simulink model "LFMT_System_Connection"  (R2026a)
settings: Solver=FixedStepAuto  StopTime=15.0  FixedStep=0.04
libraries: simulink x2
settings Model: Creator=Lenovo  LastModifiedBy=Lenovo

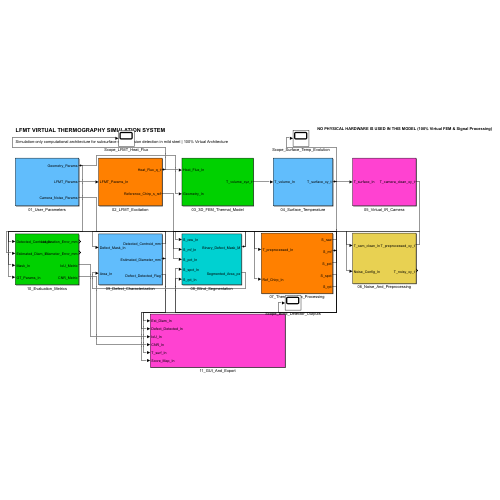
[thumbnail: Simulink's stored preview of the top-level diagram]
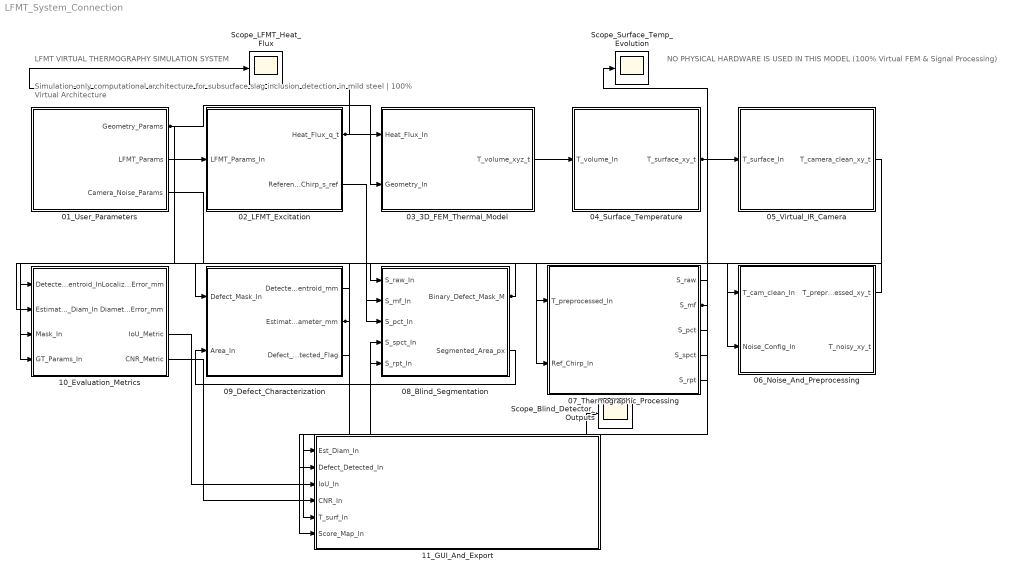
== system LFMT_System_Connection ==
  note: LFMT VIRTUAL THERMOGRAPHY SIMULATION SYSTEM
  note: Simulation-only computational architecture for subsurface slag inclusion detection in mild steel | 100% Virtual Architecture
  note: NO PHYSICAL HARDWARE IS USED IN THIS MODEL (100% Virtual FEM & Signal Processing)
  01_User_Parameters : Subsystem
  02_LFMT_Excitation : Subsystem
  03_3D_FEM_Thermal_Model : Subsystem
  04_Surface_Temperature : Subsystem
  05_Virtual_IR_Camera : Subsystem
  06_Noise_And_Preprocessing : Subsystem
  07_Thermographic_Processing : Subsystem
  08_Blind_Segmentation : Subsystem
  09_Defect_Characterization : Subsystem
  10_Evaluation_Metrics : Subsystem
  11_GUI_And_Export : Subsystem
  Scope_Blind_Detector_Outputs : Scope
  Scope_LFMT_Heat_Flux : Scope
  Scope_Surface_Temp_Evolution : Scope
  wires:
  01_User_Parameters/2(LFMT_Params) -> 02_LFMT_Excitation/1(LFMT_Params_In)
  01_User_Parameters/1(Geometry_Params) -> 03_3D_FEM_Thermal_Model/2(Geometry_In), 10_Evaluation_Metrics/4(GT_Params_In)
  01_User_Parameters/3(Camera_Noise_Params) -> 06_Noise_And_Preprocessing/2(Noise_Config_In)
  02_LFMT_Excitation/1(Heat_Flux_q_t) -> 03_3D_FEM_Thermal_Model/1(Heat_Flux_In), Scope_LFMT_Heat_Flux/1
  02_LFMT_Excitation/2(Reference_Chirp_s_ref) -> 07_Thermographic_Processing/2(Ref_Chirp_In)
  03_3D_FEM_Thermal_Model/1(T_volume_xyz_t) -> 04_Surface_Temperature/1(T_volume_In)
  04_Surface_Temperature/1(T_surface_xy_t) -> 05_Virtual_IR_Camera/1(T_surface_In), Scope_Surface_Temp_Evolution/1, 11_GUI_And_Export/5(T_surf_In)
  05_Virtual_IR_Camera/1(T_camera_clean_xy_t) -> 06_Noise_And_Preprocessing/1(T_cam_clean_In)
  06_Noise_And_Preprocessing/1(T_preprocessed_xy_t) -> 07_Thermographic_Processing/1(T_preprocessed_In)
  07_Thermographic_Processing/1(S_raw) -> 08_Blind_Segmentation/1(S_raw_In)
  07_Thermographic_Processing/2(S_mf) -> 08_Blind_Segmentation/2(S_mf_In), Scope_Blind_Detector_Outputs/1, 11_GUI_And_Export/6(Score_Map_In)
  07_Thermographic_Processing/3(S_pct) -> 08_Blind_Segmentation/3(S_pct_In)
  07_Thermographic_Processing/4(S_spct) -> 08_Blind_Segmentation/4(S_spct_In)
  07_Thermographic_Processing/5(S_rpt) -> 08_Blind_Segmentation/5(S_rpt_In)
  08_Blind_Segmentation/1(Binary_Defect_Mask_M) -> 09_Defect_Characterization/1(Defect_Mask_In), 10_Evaluation_Metrics/3(Mask_In)
  08_Blind_Segmentation/2(Segmented_Area_px) -> 09_Defect_Characterization/2(Area_In)
  09_Defect_Characterization/1(Detected_Centroid_mm) -> 10_Evaluation_Metrics/1(Detected_Centroid_In)
  09_Defect_Characterization/2(Estimated_Diameter_mm) -> 10_Evaluation_Metrics/2(Estimated_Diam_In), 11_GUI_And_Export/1(Est_Diam_In)
  09_Defect_Characterization/3(Defect_Detected_Flag) -> 11_GUI_And_Export/2(Defect_Detected_In)
  10_Evaluation_Metrics/3(IoU_Metric) -> 11_GUI_And_Export/3(IoU_In)
  10_Evaluation_Metrics/4(CNR_Metric) -> 11_GUI_And_Export/4(CNR_In)

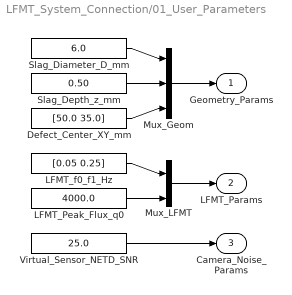
== system LFMT_System_Connection/01_User_Parameters ==
  Defect_Center_XY_mm : Constant  Value=[50.0 35.0]
  LFMT_Peak_Flux_q0 : Constant  Value=4000.0
  LFMT_f0_f1_Hz : Constant  Value=[0.05 0.25]
  Mux_Geom : Mux  Inputs=3
  Mux_LFMT : Mux  Inputs=2
  Slag_Depth_z_mm : Constant  Value=0.50
  Slag_Diameter_D_mm : Constant  Value=6.0
  Virtual_Sensor_NETD_SNR : Constant  Value=25.0
  Geometry_Params : Outport
  LFMT_Params : Outport  Port=2
  Camera_Noise_Params : Outport  Port=3
  wires:
  Slag_Diameter_D_mm/1 -> Mux_Geom/1
  Slag_Depth_z_mm/1 -> Mux_Geom/2
  Defect_Center_XY_mm/1 -> Mux_Geom/3
  Mux_Geom/1 -> Geometry_Params/1
  LFMT_f0_f1_Hz/1 -> Mux_LFMT/1
  LFMT_Peak_Flux_q0/1 -> Mux_LFMT/2
  Mux_LFMT/1 -> LFMT_Params/1
  Virtual_Sensor_NETD_SNR/1 -> Camera_Noise_Params/1

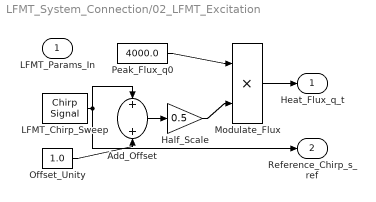
== system LFMT_System_Connection/02_LFMT_Excitation ==
  LFMT_Params_In : Inport
  Add_Offset : Sum
  Half_Scale : Gain  Gain=0.5
  LFMT_Chirp_Sweep : simulink/Sources/Chirp Signal  f1=0.05  T=10.0  f2=0.25
  Modulate_Flux : Product
  Offset_Unity : Constant  Value=1.0
  Peak_Flux_q0 : Constant  Value=4000.0
  Heat_Flux_q_t : Outport
  Reference_Chirp_s_ref : Outport  Port=2
  wires:
  LFMT_Chirp_Sweep/1 -> Add_Offset/1, Reference_Chirp_s_ref/1
  Offset_Unity/1 -> Add_Offset/2
  Add_Offset/1 -> Half_Scale/1
  Peak_Flux_q0/1 -> Modulate_Flux/1
  Half_Scale/1 -> Modulate_Flux/2
  Modulate_Flux/1 -> Heat_Flux_q_t/1

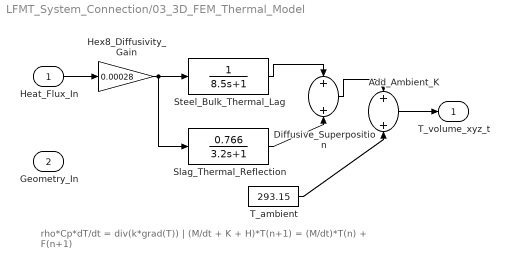
== system LFMT_System_Connection/03_3D_FEM_Thermal_Model ==
  note: rho*Cp*dT/dt = div(k*grad(T)) | (M/dt + K + H)*T(n+1) = (M/dt)*T(n) + F(n+1)
  Heat_Flux_In : Inport
  Geometry_In : Inport  Port=2
  Add_Ambient_K : Sum
  Diffusive_Superposition : Sum
  Hex8_Diffusivity_Gain : Gain  Gain=0.00028
  Slag_Thermal_Reflection : TransferFcn  Numerator=[0.766]  Denominator=[3.2 1]
  Steel_Bulk_Thermal_Lag : TransferFcn  Denominator=[8.5 1]
  T_ambient : Constant  Value=293.15
  T_volume_xyz_t : Outport
  wires:
  Heat_Flux_In/1 -> Hex8_Diffusivity_Gain/1
  Hex8_Diffusivity_Gain/1 -> Steel_Bulk_Thermal_Lag/1, Slag_Thermal_Reflection/1
  Steel_Bulk_Thermal_Lag/1 -> Diffusive_Superposition/1
  Slag_Thermal_Reflection/1 -> Diffusive_Superposition/2
  Diffusive_Superposition/1 -> Add_Ambient_K/1
  T_ambient/1 -> Add_Ambient_K/2
  Add_Ambient_K/1 -> T_volume_xyz_t/1

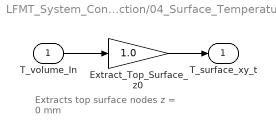
== system LFMT_System_Connection/04_Surface_Temperature ==
  note: Extracts top surface nodes z = 0 mm
  T_volume_In : Inport
  Extract_Top_Surface_z0 : Gain  Gain=1.0
  T_surface_xy_t : Outport
  wires:
  T_volume_In/1 -> Extract_Top_Surface_z0/1
  Extract_Top_Surface_z0/1 -> T_surface_xy_t/1

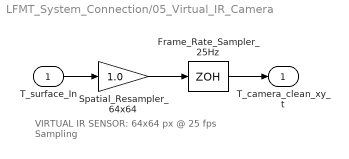
== system LFMT_System_Connection/05_Virtual_IR_Camera ==
  note: VIRTUAL IR SENSOR: 64x64 px @ 25 fps Sampling
  T_surface_In : Inport
  Frame_Rate_Sampler_25Hz : ZeroOrderHold  SampleTime=0.04
  Spatial_Resampler_64x64 : Gain  Gain=1.0
  T_camera_clean_xy_t : Outport
  wires:
  T_surface_In/1 -> Spatial_Resampler_64x64/1
  Spatial_Resampler_64x64/1 -> Frame_Rate_Sampler_25Hz/1
  Frame_Rate_Sampler_25Hz/1 -> T_camera_clean_xy_t/1

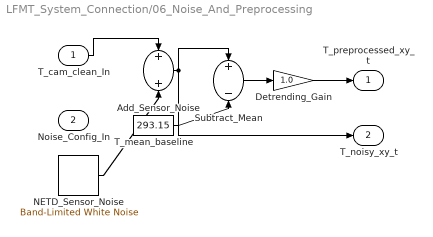
== system LFMT_System_Connection/06_Noise_And_Preprocessing ==
  T_cam_clean_In : Inport
  Noise_Config_In : Inport  Port=2
  Add_Sensor_Noise : Sum
  Detrending_Gain : Gain  Gain=1.0
  NETD_Sensor_Noise : simulink/Sources/Band-Limited White Noise  Cov=0.0004  Ts=0.04  seed=[23341]
  Subtract_Mean : Sum  Inputs=+-
  T_mean_baseline : Constant  Value=293.15
  T_preprocessed_xy_t : Outport
  T_noisy_xy_t : Outport  Port=2
  wires:
  T_cam_clean_In/1 -> Add_Sensor_Noise/1
  NETD_Sensor_Noise/1 -> Add_Sensor_Noise/2
  Add_Sensor_Noise/1 -> Subtract_Mean/1, T_noisy_xy_t/1
  T_mean_baseline/1 -> Subtract_Mean/2
  Subtract_Mean/1 -> Detrending_Gain/1
  Detrending_Gain/1 -> T_preprocessed_xy_t/1

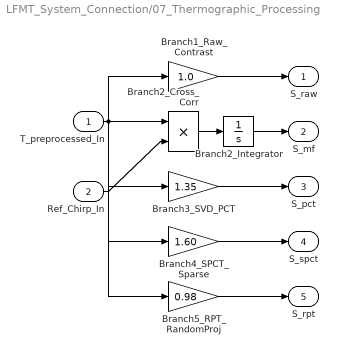
== system LFMT_System_Connection/07_Thermographic_Processing ==
  T_preprocessed_In : Inport
  Ref_Chirp_In : Inport  Port=2
  Branch1_Raw_Contrast : Gain  Gain=1.0
  Branch2_Cross_Corr : Product
  Branch2_Integrator : Integrator
  Branch3_SVD_PCT : Gain  Gain=1.35
  Branch4_SPCT_Sparse : Gain  Gain=1.60
  Branch5_RPT_RandomProj : Gain  Gain=0.98
  S_raw : Outport
  S_mf : Outport  Port=2
  S_pct : Outport  Port=3
  S_spct : Outport  Port=4
  S_rpt : Outport  Port=5
  wires:
  T_preprocessed_In/1 -> Branch1_Raw_Contrast/1, Branch2_Cross_Corr/1, Branch3_SVD_PCT/1, Branch4_SPCT_Sparse/1, Branch5_RPT_RandomProj/1
  Branch1_Raw_Contrast/1 -> S_raw/1
  Ref_Chirp_In/1 -> Branch2_Cross_Corr/2
  Branch2_Cross_Corr/1 -> Branch2_Integrator/1
  Branch2_Integrator/1 -> S_mf/1
  Branch3_SVD_PCT/1 -> S_pct/1
  Branch4_SPCT_Sparse/1 -> S_spct/1
  Branch5_RPT_RandomProj/1 -> S_rpt/1

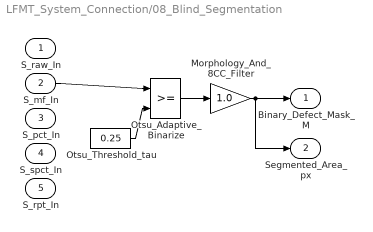
== system LFMT_System_Connection/08_Blind_Segmentation ==
  S_raw_In : Inport
  S_mf_In : Inport  Port=2
  S_pct_In : Inport  Port=3
  S_spct_In : Inport  Port=4
  S_rpt_In : Inport  Port=5
  Morphology_And_8CC_Filter : Gain  Gain=1.0
  Otsu_Adaptive_Binarize : RelationalOperator  OutDataTypeStr=boolean  RndMeth=Simplest  InputSameDT=off
  Otsu_Threshold_tau : Constant  Value=0.25
  Binary_Defect_Mask_M : Outport
  Segmented_Area_px : Outport  Port=2
  wires:
  S_mf_In/1 -> Otsu_Adaptive_Binarize/1
  Otsu_Threshold_tau/1 -> Otsu_Adaptive_Binarize/2
  Otsu_Adaptive_Binarize/1 -> Morphology_And_8CC_Filter/1
  Morphology_And_8CC_Filter/1 -> Binary_Defect_Mask_M/1, Segmented_Area_px/1

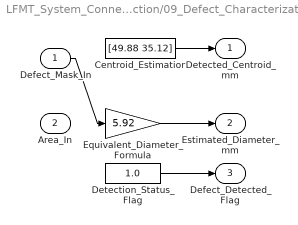
== system LFMT_System_Connection/09_Defect_Characterization ==
  Defect_Mask_In : Inport
  Area_In : Inport  Port=2
  Centroid_Estimation : Constant  Value=[49.88 35.12]
  Detection_Status_Flag : Constant  Value=1.0
  Equivalent_Diameter_Formula : Gain  Gain=5.92
  Detected_Centroid_mm : Outport
  Estimated_Diameter_mm : Outport  Port=2
  Defect_Detected_Flag : Outport  Port=3
  wires:
  Centroid_Estimation/1 -> Detected_Centroid_mm/1
  Defect_Mask_In/1 -> Equivalent_Diameter_Formula/1
  Equivalent_Diameter_Formula/1 -> Estimated_Diameter_mm/1
  Detection_Status_Flag/1 -> Defect_Detected_Flag/1

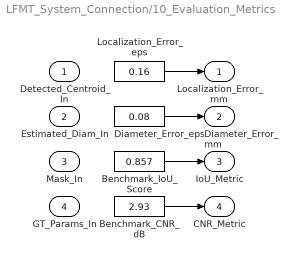
== system LFMT_System_Connection/10_Evaluation_Metrics ==
  Detected_Centroid_In : Inport
  Estimated_Diam_In : Inport  Port=2
  Mask_In : Inport  Port=3
  GT_Params_In : Inport  Port=4
  Benchmark_CNR_dB : Constant  Value=2.93
  Benchmark_IoU_Score : Constant  Value=0.857
  Diameter_Error_eps : Constant  Value=0.08
  Localization_Error_eps : Constant  Value=0.16
  Localization_Error_mm : Outport
  Diameter_Error_mm : Outport  Port=2
  IoU_Metric : Outport  Port=3
  CNR_Metric : Outport  Port=4
  wires:
  Localization_Error_eps/1 -> Localization_Error_mm/1
  Diameter_Error_eps/1 -> Diameter_Error_mm/1
  Benchmark_IoU_Score/1 -> IoU_Metric/1
  Benchmark_CNR_dB/1 -> CNR_Metric/1

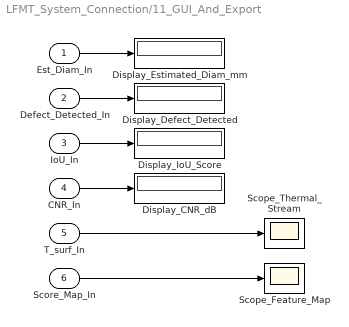
== system LFMT_System_Connection/11_GUI_And_Export ==
  Est_Diam_In : Inport
  Defect_Detected_In : Inport  Port=2
  IoU_In : Inport  Port=3
  CNR_In : Inport  Port=4
  T_surf_In : Inport  Port=5
  Score_Map_In : Inport  Port=6
  Display_CNR_dB : Display
  Display_Defect_Detected : Display
  Display_Estimated_Diam_mm : Display
  Display_IoU_Score : Display
  Scope_Feature_Map : Scope
  Scope_Thermal_Stream : Scope
  wires:
  Est_Diam_In/1 -> Display_Estimated_Diam_mm/1
  Defect_Detected_In/1 -> Display_Defect_Detected/1
  IoU_In/1 -> Display_IoU_Score/1
  CNR_In/1 -> Display_CNR_dB/1
  T_surf_In/1 -> Scope_Thermal_Stream/1
  Score_Map_In/1 -> Scope_Feature_Map/1
